simulink model "LW_ctrl_241029_1"  (R2024b)
settings: Solver=ode4  StartTime=0.0  StopTime=inf  FixedStep=0.005  RelTol=1e-3  EnableMultiTasking=on
StartFcn:
  | %timestart = cputime;
StopFcn:
  | %dt = cputime - timestart
undefined symbols (not defined in the file or in its folder): AttCtrl_cycle, ControlMode, DEG2RAD, Earth, FlightMode, LW_ACRO_P_MAX, LW_ACRO_R_MAX, LW_ACRO_Y_MAX, LW_AERO_C0, LW_AERO_C1, LW_AERO_Y0, LW_ANGLE, LW_DMZ0, LW_DMZ_MIN, LW_LAT_CIRCLE, LW_MAN_PITCH_MAX, LW_MAN_ROLL_MAX, LW_MASS, LW_OB_CIRCLE_R, LW_OB_CIRCLE_V, LW_OB_CIRCLE_W, LW_OB_TYPE, LW_REX_YAW, LW_SERVOL_MAX, LW_SERVOR_MAX, LW_TEST_DTXY, LW_TEST_DTZ, LW_THR_HOVER, LW_WZ_MAX, LW_X_ACCEL_MAX, LW_X_ACCEL_MIN, LW_X_FF, LW_X_JERK_MAX, LW_X_P, LW_X_VEL_MAX, LW_Y_ACCEL_MAX, LW_Y_ACCEL_MIN, LW_Y_FF, LW_Y_JERK_MAX, LW_Y_P, LW_Y_VEL_MAX, LW_YAW_KAD, LW_YAW_KAP, LW_Z_ACCEL_LOW, LW_Z_ACCEL_UP, LW_Z_FF, LW_Z_JERK_MAX, LW_Z_P, LW_Z_VEL_MAX_UP, Map_xoffset, Map_yoffset, Map_zoffset, MAX_wdotx, MAX_wdoty, MAX_wdotz, Mixer_cycle, ModelParam_AccelMax, ModelParam_DelayAtt, ModelParam_DelayOmega, ModelParam_DelayPos ... (+59)
libraries: pixhawk_slib_uORB_RW x15, simulink x7, slpidlib x6, dspfdesign x6, dspstat3 x5, aerolibnav x4, pixhawk_slib_sensors_actuators x3, aerolibtransform2 x3, etargetslib x2, pixhawk_slib_rfly x1, aerolibatmos2 x1, slrealtimeiplib x1
(part 4 of 6)

== system LW_ctrl_241029_1/Output/OutputSelect/Sim/Lifting Body Airframe/Estimator/Subsystem ==
  vehicle_states : Inport
  environment_states : Inport  Port=2
  Bus Selector : BusSelector  OutputSignals=Pe,Ve,wb,Vb,DCMeb,Euler,q,Ab,Abe,dwb
  Bus Selector1 : BusSelector  OutputSignals=terrainZ,landed,mag_e,mag_dec,gravity,tempcC,airPressure,altitude,airDensity,alpha,beta,airspeed,vw_e,qbar
  Transpose : Math  Operator=transpose  SignedPower=on
  Bus Element Out : Outport  PortName=Kinematics 6DOF Bus  Element=Ve
  Out Bus Element : Outport  PortName=Kinematics 6DOF Bus  Element=Xe
  Out Bus Element1 : Outport  PortName=Kinematics 6DOF Bus  Element=Euler
  Out Bus Element2 : Outport  PortName=Kinematics 6DOF Bus  Element=DCM
  Out Bus Element3 : Outport  PortName=Kinematics 6DOF Bus  Element=Vb
  Out Bus Element4 : Outport  PortName=Kinematics 6DOF Bus  Element=Wb
  Out Bus Element6 : Outport  PortName=Kinematics 6DOF Bus  Element=Abb
  Out Bus Element8 : Outport  VectorParamsAs1DForOutWhenUnconnected=off  PortName=Kinematics 6DOF Bus  Element=Quat
  Out Bus Element20 : Outport  PortName=Kinematics 6DOF Bus  Element=Abe
  Out Bus Element21 : Outport  PortName=Kinematics 6DOF Bus  Element=dWb
  Out Bus Element5 : Outport  Port=2  PortName=Environment Model Bus  Element=mag_e
  Out Bus Element7 : Outport  Port=2  PortName=Environment Model Bus  Element=mag_dec
  Out Bus Element9 : Outport  Port=2  PortName=Environment Model Bus  Element=Altitude
  Out Bus Element10 : Outport  Port=2  PortName=Environment Model Bus  Element=landed
  Out Bus Element11 : Outport  Port=2  PortName=Environment Model Bus  Element=TempC
  Out Bus Element12 : Outport  Port=2  PortName=Environment Model Bus  Element=Vwg
  Out Bus Element13 : Outport  Port=2  PortName=Environment Model Bus  Element=AirPressure
  Out Bus Element14 : Outport  Port=2  PortName=Environment Model Bus  Element=Rho
  Out Bus Element15 : Outport  Port=2  PortName=Environment Model Bus  Element=g
  Out Bus Element16 : Outport  Port=2  PortName=Environment Model Bus  Element=alpha
  Out Bus Element17 : Outport  Port=2  PortName=Environment Model Bus  Element=beta
  Out Bus Element18 : Outport  Port=2  PortName=Environment Model Bus  Element=airspeed
  Out Bus Element19 : Outport  Port=2  PortName=Environment Model Bus  Element=qbar
  Out Bus Element22 : Outport  Port=2  PortName=Environment Model Bus  Element=TerrainZ
  wires:
  Transpose/1 -> Out Bus Element2/1
  Bus Selector1/1 -> Out Bus Element22/1  "<terrainZ>"
  Bus Selector/10 -> Out Bus Element21/1  "<dwb>"
  Bus Selector/9 -> Out Bus Element20/1  "<Abe>"
  Bus Selector1/14 -> Out Bus Element19/1  "<qbar>"
  Bus Selector1/13 -> Out Bus Element12/1  "<vw_e>"
  Bus Selector1/12 -> Out Bus Element18/1  "<airspeed>"
  Bus Selector1/11 -> Out Bus Element17/1  "<beta>"
  Bus Selector1/10 -> Out Bus Element16/1  "<alpha>"
  Bus Selector1/9 -> Out Bus Element14/1  "<airDensity>"
  Bus Selector1/8 -> Out Bus Element9/1  "<altitude>"
  Bus Selector1/6 -> Out Bus Element11/1  "<tempcC>"
  Bus Selector1/7 -> Out Bus Element13/1  "<airPressure>"
  Bus Selector1/5 -> Out Bus Element15/1  "<gravity>"
  Bus Selector1/4 -> Out Bus Element7/1  "<mag_dec>"
  Bus Selector1/3 -> Out Bus Element5/1  "<mag_e>"
  Bus Selector1/2 -> Out Bus Element10/1  "<landed>"
  environment_states/1 -> Bus Selector1/1
  Bus Selector/8 -> Out Bus Element6/1  "<Ab>"
  Bus Selector/7 -> Out Bus Element8/1  "<q>"
  Bus Selector/6 -> Out Bus Element1/1  "<Euler>"
  Bus Selector/5 -> Transpose/1  "<DCMeb>"
  Bus Selector/4 -> Out Bus Element3/1  "<Vb>"
  Bus Selector/3 -> Out Bus Element4/1  "<wb>"
  Bus Selector/2 -> Bus Element Out/1  "<Ve>"
  Bus Selector/1 -> Out Bus Element/1  "<Pe>"
  vehicle_states/1 -> Bus Selector/1

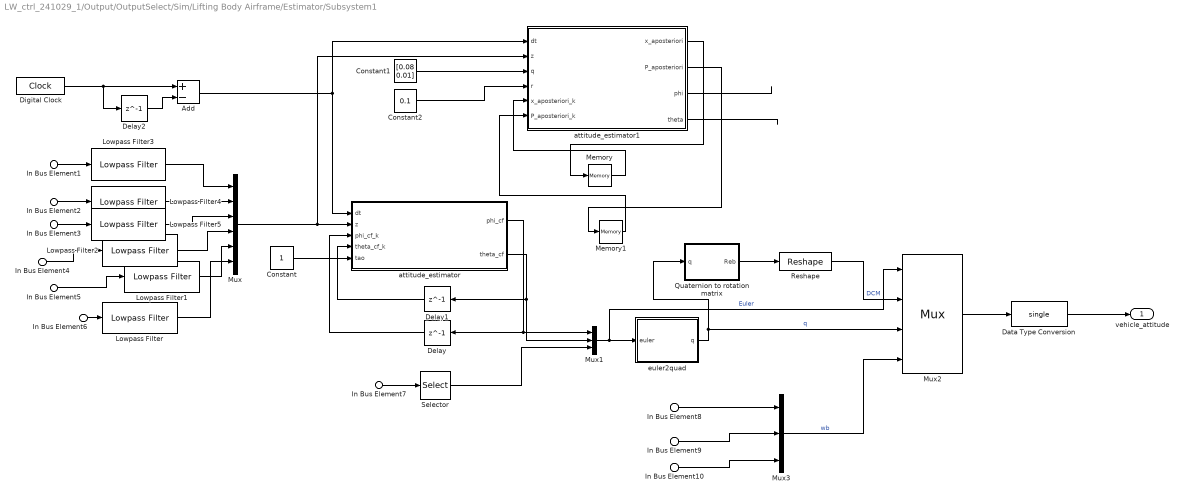
== system LW_ctrl_241029_1/Output/OutputSelect/Sim/Lifting Body Airframe/Estimator/Subsystem1 ==
  In Bus Element1 : Inport  PortName=SensorData  Element=xgyro
  In Bus Element8 : Inport  PortName=SensorData  Element=xgyro
  In Bus Element2 : Inport  PortName=SensorData  Element=ygyro
  In Bus Element9 : Inport  PortName=SensorData  Element=ygyro
  In Bus Element3 : Inport  PortName=SensorData  Element=zgyro
  In Bus Element10 : Inport  PortName=SensorData  Element=zgyro
  In Bus Element4 : Inport  PortName=SensorData  Element=xacc
  In Bus Element5 : Inport  PortName=SensorData  Element=yacc
  In Bus Element6 : Inport  PortName=SensorData  Element=zacc
  In Bus Element7 : Inport  Port=2  PortName=Kinematics 6DOF Bus  Element=Euler
  Add : Sum  Inputs=+-
  Constant : Constant
  Constant1 : Constant  Value=[0.08 0.01]
  Constant2 : Constant  Value=0.1
  Data Type Conversion : DataTypeConversion  OutDataTypeStr=single  SaturateOnIntegerOverflow=off  RndMeth=Floor
  Delay : Delay  DelayLength=1  InitialCondition=0
  Delay1 : Delay  DelayLength=1  InitialCondition=0
  Delay2 : Delay  DelayLength=1  InitialCondition=0
  Digital Clock : DigitalClock  SampleTime=0.001
  Lowpass Filter{,1..5} (6 alike) : dspfdesign/Lowpass Filter  FilterType=FIR  DesignForMinimumOrder=on  FilterOrder=50  PassbandFrequency=10  StopbandFrequency=40  PassbandRipple=0.1  StopbandAttenuation=80  SampleRateMode=Specify on dialog  SampleRate=1000  SimulateUsing=Interpreted execution  roundingMode=Floor  coeffsDataTypeStr=fixdt(1,16)
  Memory : Memory  InitialCondition=[0, 0, 0, 0, 0, -1]
  Memory1 : Memory  InitialCondition=eye(6, 6)*100
  Mux : Mux  Inputs=6
  Mux1 : Mux  Inputs=3
  Mux2 : Mux
      settings: DisplayOption=signals
  Mux3 : Mux  Inputs=3
  Quaternion to rotation matrix : MATLAB Function
  Reshape : Reshape
  Selector : Selector  InputPortWidth=3  IndexOptions=Index vector (dialog)  Indices=[ 3]  OutputSizes=1
  attitude_estimator : MATLAB Function  TreatAsAtomicUnit=on
  attitude_estimator1 : MATLAB Function  TreatAsAtomicUnit=on
  euler2quad : MATLAB Function
  vehicle_attitude : Outport
  wires:
  Constant/1 -> attitude_estimator/5(tao)
  Delay1/1 -> attitude_estimator/4(theta_cf_k)
  Delay/1 -> attitude_estimator/3(phi_cf_k)
  Mux/1 -> attitude_estimator1/2(z), attitude_estimator/2(z)
  In Bus Element1/1 -> Lowpass Filter3/1
  In Bus Element2/1 -> Lowpass Filter4/1
  In Bus Element3/1 -> Lowpass Filter5/1
  In Bus Element4/1 -> Lowpass Filter2/1
  In Bus Element5/1 -> Lowpass Filter1/1
  In Bus Element6/1 -> Lowpass Filter/1
  attitude_estimator/1(phi_cf) -> Mux1/1, Delay/1
  attitude_estimator/2(theta_cf) -> Mux1/2, Delay1/1
  Digital Clock/1 -> Add/1, Delay2/1
  Delay2/1 -> Add/2
  Add/1 -> attitude_estimator/1(dt), attitude_estimator1/1(dt)
  In Bus Element7/1 -> Selector/1
  Selector/1 -> Mux1/3
  Mux1/1 -> Mux2/1, euler2quad/1(euler)  "Euler"
  euler2quad/1(q) -> Quaternion to rotation matrix/1(q), Mux2/3  "q"
  Quaternion to rotation matrix/1(Reb) -> Reshape/1
  Reshape/1 -> Mux2/2  "DCM"
  In Bus Element8/1 -> Mux3/1
  In Bus Element9/1 -> Mux3/2
  In Bus Element10/1 -> Mux3/3
  Mux3/1 -> Mux2/4  "wb"
  Mux2/1 -> Data Type Conversion/1
  Data Type Conversion/1 -> vehicle_attitude/1
  attitude_estimator1/1(x_aposteriori) -> Memory/1
  Memory/1 -> attitude_estimator1/5(x_aposteriori_k)
  attitude_estimator1/2(P_aposteriori) -> Memory1/1
  Memory1/1 -> attitude_estimator1/6(P_aposteriori_k)
  attitude_estimator1/3(phi) -> ?
  attitude_estimator1/4(theta) -> ?
  Constant1/1 -> attitude_estimator1/3(q)
  Constant2/1 -> attitude_estimator1/4(r)
  Lowpass Filter/1 -> Mux/6
  Lowpass Filter1/1 -> Mux/5
  Lowpass Filter2/1 -> Mux/4
  Lowpass Filter3/1 -> Mux/1
  Lowpass Filter4/1 -> Mux/2
  Lowpass Filter5/1 -> Mux/3

== system LW_ctrl_241029_1/Output/OutputSelect/Sim/Lifting Body Airframe/Estimator/Subsystem2 ==
  In Bus Element1 : Inport  PortName=SensorData  Element=xgyro
  In Bus Element2 : Inport  PortName=SensorData  Element=ygyro
  In Bus Element3 : Inport  PortName=SensorData  Element=zgyro
  In Bus Element4 : Inport  PortName=SensorData  Element=xacc
  In Bus Element5 : Inport  PortName=SensorData  Element=yacc
  In Bus Element6 : Inport  PortName=SensorData  Element=zacc
  Data Type Conversion : DataTypeConversion  OutDataTypeStr=single  SaturateOnIntegerOverflow=off  RndMeth=Floor
  Mux : Mux  Inputs=6
  imu : Outport
  wires:
  In Bus Element3/1 -> Mux/3
  In Bus Element2/1 -> Mux/2
  In Bus Element1/1 -> Mux/1
  In Bus Element4/1 -> Mux/4
  In Bus Element5/1 -> Mux/5
  In Bus Element6/1 -> Mux/6
  Data Type Conversion/1 -> imu/1
  Mux/1 -> Data Type Conversion/1

== system LW_ctrl_241029_1/Output/OutputSelect/Sim/Lifting Body Airframe/To Unreal/pack ==
  note: struct SOut2Simulator
      | {
      | int copterID; //飞机ID
      | int vehicleType; //飞机构型
      | double runnedTime; //仿真时间
      | float VelE[3]; //NED地球系速度
      | float PosE[3]; //NED地球系位置
      | float AngEuler[3]; //欧拉角
      | float AngQuatern[4]; //四元数
      | float MotorRPMS[8]; //电机转速RPM
      | float AccB[3]; //机体轴加速度
      | float RateB[3]; //机体轴角速度
      | double PosGPS[3]; //地球GPS经纬高
      | }
      |
      | //SOut2Simulator的定义与Simulink里面新加的MavVehileInfo结构体完全一致
      | //可以直接对新的simulink模型的MavVehile3DInfo输出口数据进行打包
      | //两个结构体的长度都是152
      | sizeof(SOut2Simulator) = sizeof(MavVehileInfo) = 152
      |
      | 打包封装的结构体为
      | typedef struct _netDataShort
      | {
      | TargetType tg; //这里目前随便填，写1即可 uint32
      | int len; //这个长度为传输结构体长度，目前是152
      | char payload[192]; //这里面前152位存放了SOut2Simulator结构体数据，后面的40位保留
      | }netDataShort;
      |
      | //UDP包的总长度为200
      | sizeof(netDataShort) = 200
      |
      | //发送的UDP端口号为：20010
  copterID : Inport  PortDimensions=1
  vehicleType : Inport  Port=2  PortDimensions=1
  runnedTime : Inport  Port=3  PortDimensions=1
  "VelE " : Inport  Port=4  PortDimensions=3
  PosE : Inport  Port=5  PortDimensions=3
  AngEuler : Inport  Port=6  PortDimensions=3
  AngQuatern : Inport  Port=7  PortDimensions=4
  MotorRPMS : Inport  Port=8  PortDimensions=8
  AccB : Inport  Port=9  PortDimensions=3
  RateB : Inport  Port=10  PortDimensions=3
  PosGPS : Inport  Port=11  PortDimensions=3
  Data Type Conversion : DataTypeConversion  OutDataTypeStr=uint32  SaturateOnIntegerOverflow=off  RndMeth=Floor
  Data Type Conversion1 : DataTypeConversion  OutDataTypeStr=int32  SaturateOnIntegerOverflow=off  RndMeth=Floor
  Data Type Conversion2 : DataTypeConversion  OutDataTypeStr=int32  SaturateOnIntegerOverflow=off  RndMeth=Floor
  Data Type Conversion3 : DataTypeConversion  OutDataTypeStr=int32  SaturateOnIntegerOverflow=off  RndMeth=Floor
  Data Type Conversion4 : DataTypeConversion  OutDataTypeStr=double  SaturateOnIntegerOverflow=off  RndMeth=Floor
  Data Type Conversion5 : DataTypeConversion  OutDataTypeStr=single  SaturateOnIntegerOverflow=off  RndMeth=Floor
  Data Type Conversion6 : DataTypeConversion  OutDataTypeStr=double  SaturateOnIntegerOverflow=off  RndMeth=Floor
  Data Type Conversion7 : DataTypeConversion  OutDataTypeStr=double  SaturateOnIntegerOverflow=off  RndMeth=Floor
  Mux : Mux  Inputs=2
  Mux1 : Mux  Inputs=7
  Mux2 : Mux  Inputs=2
  Package Head : etargetslib/Byte Pack  datatypes={'uint32','int32'}  byteAlign=4
  PayLoad : etargetslib/Byte Pack  datatypes={'int32','double','single','double','double'}  byteAlign=8
  TargetType : Constant  OutDataTypeStr=Inherit: Inherit via back propagation
  len : Constant  Value=152  OutDataTypeStr=Inherit: Inherit via back propagation
  reserve : Constant  Value=[0 0 0 0 0]  OutDataTypeStr=double
  toUnReal : Outport  VectorParamsAs1DForOutWhenUnconnected=off
  wires:
  Data Type Conversion7/1 -> PayLoad/5
  Data Type Conversion4/1 -> PayLoad/2
  Data Type Conversion3/1 -> Mux2/2
  Data Type Conversion/1 -> Package Head/1
  Data Type Conversion6/1 -> PayLoad/4
  Data Type Conversion1/1 -> Package Head/2
  Data Type Conversion2/1 -> Mux2/1
  Data Type Conversion5/1 -> PayLoad/3
  AngEuler/1 -> Mux1/3
  Mux2/1 -> PayLoad/1
  reserve/1 -> Data Type Conversion7/1
  TargetType/1 -> Data Type Conversion/1
  PosE/1 -> Mux1/2
  vehicleType/1 -> Data Type Conversion3/1
  len/1 -> Data Type Conversion1/1
  copterID/1 -> Data Type Conversion2/1
  AngQuatern/1 -> Mux1/4
  MotorRPMS/1 -> Mux1/5
  Mux/1 -> toUnReal/1
  AccB/1 -> Mux1/6
  Package Head/1 -> Mux/1
  PosGPS/1 -> Data Type Conversion6/1
  Mux1/1 -> Data Type Conversion5/1
  "VelE "/1 -> Mux1/1
  PayLoad/1 -> Mux/2
  RateB/1 -> Mux1/7
  runnedTime/1 -> Data Type Conversion4/1

== system LW_ctrl_241029_1/rc_receive/manual_ctrl_in/Sim/Simulate ref/commandMapping/command2pwm ==
  rates_ref : Inport
  ctrl_mode : Inport  Port=2
  euler_ref : Inport  Port=3
  vel_ref : Inport  Port=4
  throttle : Inport  Port=5
  delta : Inport  Port=6
  Merge : Merge  Inputs=5
  Switch Case : SwitchCase  CaseConditions={ControlMode.MANUAL,ControlMode.ACRO, ControlMode.STABILIZED, ControlMode.ALTITUDE,ControlMode.POSITION}
  Terminator : Terminator
  acro : Subsystem  TreatAsAtomicUnit=on
  altitude : Subsystem  TreatAsAtomicUnit=on
  euler_ref1 : InportShadow  Port=3
  man : Subsystem  TreatAsAtomicUnit=on
  position : Subsystem  TreatAsAtomicUnit=on
  rates_r_ref : InportShadow
  rates_r_ref1 : InportShadow
  rates_r_ref2 : InportShadow
  stabilized : Subsystem  TreatAsAtomicUnit=on
  throttle1 : InportShadow  Port=5
  vel_ref1 : InportShadow  Port=4
  manual_ref : Outport
  wires:
  Switch Case/4 -> altitude/Action
  Switch Case/3 -> stabilized/Action
  ctrl_mode/1 -> Switch Case/1
  rates_ref/1 -> acro/1(rc_input)
  altitude/1(altitude_ref) -> Merge/4
  Switch Case/2 -> acro/Action
  stabilized/1(stabilizd_ref) -> Merge/3
  Switch Case/5 -> position/Action
  throttle/1 -> acro/2(throttle)
  euler_ref/1 -> stabilized/1(euler_ref)
  throttle1/1 -> stabilized/2(throttle)
  vel_ref/1 -> altitude/3(vel_ref)
  rates_r_ref/1 -> stabilized/3(rates_r_ref)
  rates_r_ref1/1 -> altitude/2(rates_r_ref)
  vel_ref1/1 -> position/1(vel_ref)
  rates_r_ref2/1 -> position/2(rates_r_ref)
  euler_ref1/1 -> altitude/1(euler_ref)
  position/1(position_ref) -> Merge/5
  acro/1(acro_ref) -> Merge/2
  Switch Case/6 -> Terminator/1
  Merge/1 -> manual_ref/1
  delta/1 -> man/1(delta)
  Switch Case/1 -> man/Action
  man/1(delta_ref) -> Merge/1

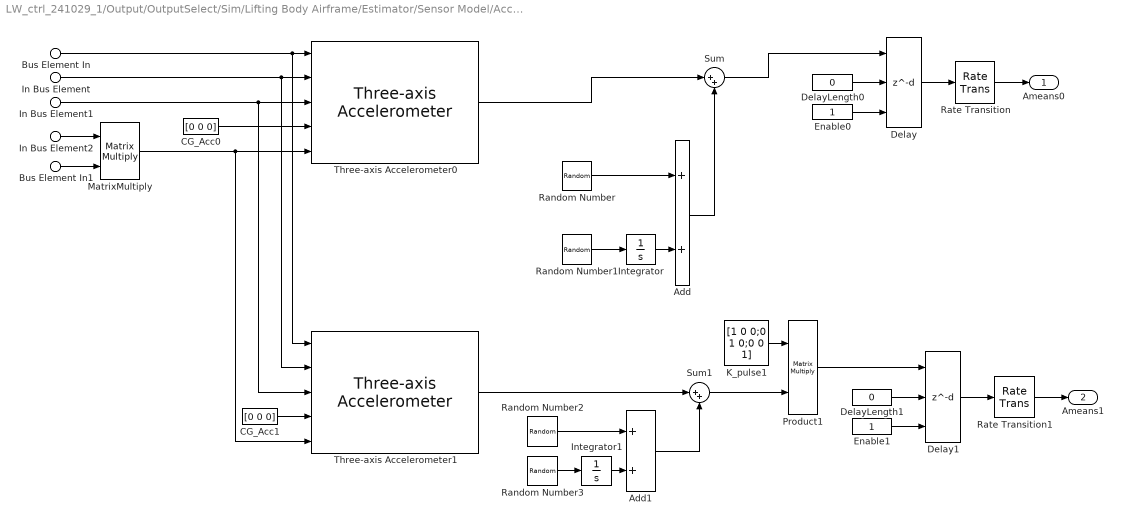
== system LW_ctrl_241029_1/Output/OutputSelect/Sim/Lifting Body Airframe/Estimator/Sensor Model/Accelerometer Hub ==
  Bus Element In1 : Inport  PortName=Environment Model Bus  Element=g
  Bus Element In : Inport  Port=2  PortName=Kinematics 6DOF Bus  Element=Abe
  In Bus Element : Inport  Port=2  PortName=Kinematics 6DOF Bus  Element=Wb
  In Bus Element1 : Inport  Port=2  PortName=Kinematics 6DOF Bus  Element=dWb
  In Bus Element2 : Inport  Port=2  PortName=Kinematics 6DOF Bus  Element=DCM
  Add : Sum
  Add1 : Sum
  CG_Acc0 : Constant  Value=[0 0 0]
  CG_Acc1 : Constant  Value=[0 0 0]
  Delay : Delay  DelayLengthSource=Input port  ShowEnablePort=on
      settings: InputPortMap=u0,p1,e6
  Delay1 : Delay  DelayLengthSource=Input port  ShowEnablePort=on
      settings: InputPortMap=u0,p1,e6
  DelayLength0 : Constant  Value=0
  DelayLength1 : Constant  Value=0
  Enable0 : Constant
  Enable1 : Constant
  Integrator : Integrator
  Integrator1 : Integrator
  K_pulse1 : Constant  Value=[1 0 0;0 1 0;0 0 1]
  MatrixMultiply : Product  Multiplication=Matrix(*)
  Product1 : Product  Multiplication=Matrix(*)
  Random Number : RandomNumber  Variance=ModelParam_noiseAccelNa  Seed=ModelParam_noiseAccelNaSeed  SampleTime=0.004
  Random Number1 : RandomNumber  Variance=ModelParam_noiseAccelBa  Seed=ModelParam_noiseAccelBaSeed  SampleTime=0.004
  Random Number2 : RandomNumber  Mean=[0 0 0]  Variance=[0.1 0.1 0.1]  Seed=[235 341 569]  SampleTime=SampleTime
  Random Number3 : RandomNumber  Mean=[0 0 0]  Variance=[0.1 0.1 0.1]  Seed=[3341 365 597]  SampleTime=SampleTime
  Rate Transition : RateTransition
  Rate Transition1 : RateTransition
  Sum : Sum  Inputs=|++
  Sum1 : Sum  Inputs=|++
  Three-axis Accelerometer0 : aerolibnav/Three-axis Accelerometer  units=Metric (MKS)  acc=[0 0 0]  gtype=on  dtype_a=on  w_a=190  z_a=0.707  a_sf_cc=[1 0 0; 0 1 0; 0 0 1]  a_bias=[0 0 0]  a_Ts=0  a_rand=off  a_seeds=[23093 23094 23095]  a_pow=[0.001 0.001 0.001]  a_sat="[-inf  -inf  -inf  inf inf inf]"
  Three-axis Accelerometer1 : aerolibnav/Three-axis Accelerometer  units=Metric (MKS)  acc=[0 0 0]  gtype=on  dtype_a=on  w_a=190  z_a=0.707  a_sf_cc=[1 0 0; 0 1 0; 0 0 1]  a_bias=[0 0 0]  a_Ts=0  a_rand=off  a_seeds=[23093 23094 23095]  a_pow=[0.001 0.001 0.001]  a_sat="[-inf  -inf  -inf  inf inf inf]"
  Ameans0 : Outport
  Ameans1 : Outport  Port=2
  wires:
  Add/1 -> Sum/2
  Random Number1/1 -> Integrator/1
  Random Number/1 -> Add/1
  Three-axis Accelerometer0/1 -> Sum/1
  K_pulse1/1 -> Product1/1
  Product1/1 -> Delay1/1
  Sum/1 -> Delay/1
  Random Number2/1 -> Add1/1
  Integrator1/1 -> Add1/2
  Random Number3/1 -> Integrator1/1
  Add1/1 -> Sum1/2
  Sum1/1 -> Product1/2
  Integrator/1 -> Add/2
  In Bus Element2/1 -> MatrixMultiply/1
  Bus Element In/1 -> Three-axis Accelerometer0/1, Three-axis Accelerometer1/1
  In Bus Element/1 -> Three-axis Accelerometer0/2, Three-axis Accelerometer1/2
  Bus Element In1/1 -> MatrixMultiply/2
  In Bus Element1/1 -> Three-axis Accelerometer1/3, Three-axis Accelerometer0/3
  Delay1/1 -> Rate Transition1/1
  Three-axis Accelerometer1/1 -> Sum1/1
  Rate Transition1/1 -> Ameans1/1
  Enable1/1 -> Delay1/3
  DelayLength1/1 -> Delay1/2
  DelayLength0/1 -> Delay/2
  Enable0/1 -> Delay/3
  Rate Transition/1 -> Ameans0/1
  CG_Acc0/1 -> Three-axis Accelerometer0/4
  Delay/1 -> Rate Transition/1
  CG_Acc1/1 -> Three-axis Accelerometer1/4
  MatrixMultiply/1 -> Three-axis Accelerometer0/5, Three-axis Accelerometer1/5

== system LW_ctrl_241029_1/Output/OutputSelect/Sim/Lifting Body Airframe/Estimator/Sensor Model/Barometer ==
  In Bus Element : Inport  PortName=Environment Model Bus  Element=Altitude
  In Bus Element2 : Inport  PortName=Environment Model Bus  Element=TempC
  In Bus Element1 : Inport  PortName=Environment Model Bus  Element=qbar
  Add2 : Sum
  Gain : Gain  Gain=0.01
  Gain3 : Gain  Gain=0.01
  ISA Atmosphere Model : aerolibatmos2/ISA Atmosphere Model  useExtended=off  action=Warning  custom=off  viscosityOut=off  g=9.80665  gamma=1.4  R=287.0531  L=0.0065  h_trop=11000  h_strat=20000  rho0=1.225  P0=101325  T0=288.15  h0=0  S=110.4  Tref=273.15  muref=1.716e-5
  Integrator1 : Integrator
  K_pulse0 : Constant
  Product : Product
  Random Number1 : RandomNumber  Variance=ModelParam_noiseBaroNm  Seed=ModelParam_noiseBaroNmSeed  SampleTime=0.004
  Random Number2 : RandomNumber  Variance=ModelParam_noiseBaroNbm  Seed=ModelParam_noiseBaroNbmSeed  SampleTime=0.004
  Sum : Sum  Inputs=|++
  Terminator : Terminator
  Terminator1 : Terminator
  Terminator2 : Terminator
  Pressure : Outport
  diff_pressure : Outport  Port=2
  pressure_alt : Outport  Port=3  PortDimensions=1
  temperature : Outport  Port=4
  wires:
  In Bus Element1/1 -> Gain/1
  ISA Atmosphere Model/4 -> Terminator2/1
  ISA Atmosphere Model/2 -> Terminator1/1
  ISA Atmosphere Model/1 -> Terminator/1
  Random Number2/1 -> Integrator1/1
  Add2/1 -> Sum/2
  Random Number1/1 -> Add2/1
  Integrator1/1 -> Add2/2
  Gain3/1 -> Pressure/1
  Gain/1 -> diff_pressure/1
  In Bus Element2/1 -> temperature/1
  ISA Atmosphere Model/3 -> Gain3/1
  K_pulse0/1 -> Product/1
  Sum/1 -> Product/2
  In Bus Element/1 -> Sum/1
  Product/1 -> pressure_alt/1, ISA Atmosphere Model/1

== system LW_ctrl_241029_1/Output/OutputSelect/Sim/Lifting Body Airframe/Estimator/Sensor Model/GPS ==
  In Bus Element : Inport  PortName=Kinematics 6DOF Bus  Element=Xe
  In Bus Element1 : Inport  PortName=Kinematics 6DOF Bus  Element=Ve
  In Bus Element2 : Inport  PortName=Kinematics 6DOF Bus  Element=Euler
  -pi-pi---->0-2pi : MATLAB Function  TreatAsAtomicUnit=on
  BiasGain1 : Gain  Gain=0.1
  Demux : Demux  Outputs=3
  Demux1 : Demux  Outputs=3
  Flat Earth to LLA : aerolibtransform2/Flat Earth to LLA  units=Metric (MKS)  ptype=Earth (WGS84)  F=1/298.257223563  R=6378137  refPosPort=off  LL0=ModelParam_GPSLatLong  psi=0
  Gain1 : Gain  Gain=0.2*0.58
  GenCogVel : MATLAB Function  TreatAsAtomicUnit=on
  ModelParam.GPSEphFinal : Constant  Value=ModelParam_GPSEphFinal
  ModelParam.GPSEpvFinal : Constant  Value=ModelParam_GPSEpvFinal
  ModelParam.GPSSatsVisible : Constant  Value=ModelParam_GPSSatsVisible
  ModelParam_GPSFix3DFix : Constant  Value=ModelParam_GPSFix3DFix
  ModelParam_envAltitude : Constant  Value=ModelParam_envAltitude
  Mux : Mux  Inputs=2
  Mux1 : Mux  Inputs=13
  NoiseFilter1 : Subsystem
  Saturation : Saturate  UpperLimit=100000  LowerLimit=0
  Selector : Selector  InputPortWidth=3  IndexOptions=Index vector (dialog)  Indices=[3]  OutputSizes=1
  Sum : Sum  Inputs=|++
  Sum3 : Sum  Inputs=|++
  Uniform Random Number1 : UniformRandomNumber  Minimum=[-1,-1,-2]  Maximum=[1,1,2]  Seed=[1452,787,69]  SampleTime=ModelParam_noiseGPSSampTime
  Uniform Random Number4 : UniformRandomNumber  Minimum=[-1,-1,-2]  Maximum=[1,1,2]  Seed=[5445,45433,33433]  SampleTime=ModelParam_noiseGPSSampTime
  GPS : Outport
  wires:
  NoiseFilter1/1(Out1) -> Sum3/2
  BiasGain1/1 -> NoiseFilter1/1(In1)
  Uniform Random Number4/1 -> BiasGain1/1
  Sum3/1 -> GenCogVel/1(u), Demux1/1
  Saturation/1 -> Mux/2
  Gain1/1 -> Sum/2
  Uniform Random Number1/1 -> Gain1/1
  ModelParam.GPSSatsVisible/1 -> Mux1/12  "satellites_visible"
  ModelParam_GPSFix3DFix/1 -> Mux1/11  "fixtype"
  -pi-pi---->0-2pi/1(yaw360) -> Mux1/13  "headVeh"
  Selector/1 -> -pi-pi---->0-2pi/1(yaw180)
  In Bus Element2/1 -> Selector/1
  GenCogVel/2(cot) -> Mux1/7  "cog"
  GenCogVel/1(v) -> Mux1/6  "vel"
  Demux1/3 -> Mux1/10  "vd"
  Demux1/2 -> Mux1/9  "ve"
  Demux1/1 -> Mux1/8  "vn"
  In Bus Element1/1 -> Sum3/1
  Mux1/1 -> GPS/1
  ModelParam.GPSEpvFinal/1 -> Mux1/5  "epv"
  ModelParam.GPSEphFinal/1 -> Mux1/4  "eph"
  Demux/3 -> Mux1/3  "alt"
  Demux/1 -> Mux1/1  "lat"
  Demux/2 -> Mux1/2  "lon"
  Mux/1 -> Demux/1
  Flat Earth to LLA/2 -> Saturation/1
  Flat Earth to LLA/1 -> Mux/1
  Sum/1 -> Flat Earth to LLA/1
  In Bus Element/1 -> Sum/1
  ModelParam_envAltitude/1 -> Flat Earth to LLA/2

== system LW_ctrl_241029_1/Output/OutputSelect/Sim/Lifting Body Airframe/Estimator/Sensor Model/Gyroscope Hub ==
  In Bus Element : Inport  PortName=Kinematics 6DOF Bus  Element=Wb
  In Bus Element1 : Inport  PortName=Kinematics 6DOF Bus  Element=Abe
  Acceleration Conversion : aerolibnav/Three-axis Inertial Measurement Unit/Acceleration Conversion  SystemSampleTime=-1  VariantActivationTime=update diagram  AllowFlexibleInterface=on  Latency=0  AutoFrameSizeCalculation=off
  Add2 : Sum
  Delay : Delay  DelayLengthSource=Input port  ShowEnablePort=on
      settings: InputPortMap=u0,p1,e6
  DelayLength0 : Constant  Value=0
  Enable0 : Constant
  Integrator : Integrator
  Random Number : RandomNumber  Variance=ModelParam_noiseGyroNg  Seed=ModelParam_noiseGyroNgSeed  SampleTime=0.004
  Random Number1 : RandomNumber  Variance=ModelParam_noiseGyroNbg  Seed=ModelParam_noiseGyroNbgSeed  SampleTime=0.004
  Rate Transition : RateTransition
  Sum : Sum  Inputs=|++
  Three-axis Gyroscope0 : aerolibnav/Three-axis Gyroscope  dtype_g=on  w_g=190  z_g=0.707  g_sf_cc=[1 0 0; 0 1 0; 0 0 1]  g_bias=[0 0 0]  g_sen=[0 0 0]  g_Ts=0  g_rand=off  g_seeds=[23093 23094 23095]  g_pow=[0.0001 0.0001 0.0001]  g_sat="[-inf  -inf  -inf  inf inf inf]"
  Wmeans0 : Outport
  wires:
  Sum/1 -> Delay/1
  Random Number/1 -> Add2/1
  Add2/1 -> Sum/2
  Three-axis Gyroscope0/1 -> Sum/1
  Random Number1/1 -> Integrator/1
  Integrator/1 -> Add2/2
  DelayLength0/1 -> Delay/2
  Rate Transition/1 -> Wmeans0/1
  Delay/1 -> Rate Transition/1
  Enable0/1 -> Delay/3
  Acceleration Conversion/1 -> Three-axis Gyroscope0/2
  In Bus Element/1 -> Three-axis Gyroscope0/1
  In Bus Element1/1 -> Acceleration Conversion/1

== system LW_ctrl_241029_1/Output/OutputSelect/Sim/Lifting Body Airframe/Estimator/Sensor Model/Magnetometer Hub ==
  In Bus Element : Inport  PortName=Kinematics 6DOF Bus  Element=DCM
  In Bus Element1 : Inport  Port=2  PortName=Environment Model Bus  Element=mag_e
  In Bus Element3 : Inport  Port=2  PortName=Environment Model Bus  Element=mag_e
  Delay : Delay  DelayLengthSource=Input port  ShowEnablePort=on
      settings: InputPortMap=u0,p1,e6
  Delay1 : Delay  DelayLengthSource=Input port  ShowEnablePort=on
      settings: InputPortMap=u0,p1,e6
  DelayLength0 : Constant  Value=0
  DelayLength1 : Constant  Value=0
  Enable0 : Constant
  Enable1 : Constant
  Integrator : Integrator
  Integrator1 : Integrator
  K_m1 : Constant  Value=[1 0 0; 0 1 0; 0 0 1]
  K_m2 : Constant  Value=[1 0 0; 0 1 0; 0 0 1]
  K_pulse0 : Constant  Value=[1 0 0;0 1 0;0 0 1]
  K_pulse1 : Constant  Value=[1 0 0;0 1 0;0 0 1]
  MATLAB Function : MATLAB Function  TreatAsAtomicUnit=on
  MATLAB Function1 : MATLAB Function  TreatAsAtomicUnit=on
  Measurement bias1 : Constant  Value=[0 0 0]
  Product : Product  Multiplication=Matrix(*)
  Product1 : Product  Multiplication=Matrix(*)
  Random Number : RandomNumber  Variance=ModelParam_noiseMagNm  Seed=ModelParam_noiseMagNmSeed  SampleTime=0.004
  Random Number1 : RandomNumber  Variance=ModelParam_noiseMagNm  Seed=[45465,454534,1234232]  SampleTime=0.004
  Random Number2 : RandomNumber  Mean=[0 0 0]  Variance=[0.1 0.1 0.1]  Seed=[666 588 477]  SampleTime=0.001
  Random Number3 : RandomNumber  Mean=[0 0 0]  Variance=[0.1 0.1 0.1]  Seed=[111 222 333]  SampleTime=0.001
  Rate Transition : RateTransition
  Rate Transition1 : RateTransition
  Sum1 : Sum  Inputs=|++
  Mag_means0 : Outport
  Mag_means1 : Outport  Port=2
  wires:
  In Bus Element3/1 -> MATLAB Function1/2(mag_e)
  In Bus Element1/1 -> MATLAB Function/2(mag_e)
  Integrator/1 -> MATLAB Function/3(b_m)
  Random Number/1 -> MATLAB Function/4(n_m)
  K_m2/1 -> MATLAB Function/5(K_m)
  Measurement bias1/1 -> Sum1/2
  Sum1/1 -> MATLAB Function1/3(b_m)
  Product1/1 -> Delay1/1
  K_pulse1/1 -> Product1/1
  K_pulse0/1 -> Product/1
  Product/1 -> Delay/1
  Random Number3/1 -> Integrator1/1
  Random Number1/1 -> Integrator/1
  Rate Transition1/1 -> Mag_means1/1
  Delay1/1 -> Rate Transition1/1
  DelayLength1/1 -> Delay1/2
  Enable1/1 -> Delay1/3
  MATLAB Function1/1(Mag_means) -> Product1/2
  MATLAB Function/1(Mag_means) -> Product/2
  Enable0/1 -> Delay/3
  DelayLength0/1 -> Delay/2
  Delay/1 -> Rate Transition/1
  Rate Transition/1 -> Mag_means0/1
  Random Number2/1 -> MATLAB Function1/4(n_m)
  Integrator1/1 -> Sum1/1
  K_m1/1 -> MATLAB Function1/5(K_m)
  In Bus Element/1 -> MATLAB Function1/1(DCM), MATLAB Function/1(DCM)

== system LW_ctrl_241029_1/rc_receive/manual_ctrl_in/Sim/Simulate ref/commandMapping/command2pwm/acro ==
  rc_input : Inport
  throttle : Inport  Port=2
  Action Port : ActionPort  ActionPortLabel=case [ ACRO ]:
  Constant7 : Constant  Value=1000
  Constant8 : Constant  Value=1500
  Data Type Conversion4 : DataTypeConversion  OutDataTypeStr=single  SaturateOnIntegerOverflow=off  RndMeth=Floor
  Data Type Conversion5 : DataTypeConversion  OutDataTypeStr=single  SaturateOnIntegerOverflow=off  RndMeth=Floor
  Demux : Demux  Outputs=3
  Gain1 : Gain  Gain=1/LW_ACRO_R_MAX
  Gain10 : Gain  Gain=1/LW_ACRO_P_MAX
  Gain12 : Gain  Gain=1/LW_ACRO_Y_MAX
  Gain4 : Gain  Gain=RC1_REV
  Mux1 : Mux  Inputs=6
      settings: DisplayOption=signals
  Saturation1 : Saturate  UpperLimit=1  LowerLimit=0
  Saturation2 : Saturate  UpperLimit=1  LowerLimit=-1
  Saturation3 : Saturate  UpperLimit=1  LowerLimit=-1
  Saturation4 : Saturate  UpperLimit=1  LowerLimit=-1
  wx_deadzone_inv : MATLAB Function  TreatAsAtomicUnit=on
  wy_deadzone_inv : MATLAB Function  TreatAsAtomicUnit=on
  wz_deadzone_inv : MATLAB Function  TreatAsAtomicUnit=on
  acro_ref : Outport
  wires:
  rc_input/1 -> Demux/1
  Demux/1 -> Gain1/1
  Gain1/1 -> wy_deadzone_inv/1(u)
  Gain10/1 -> wx_deadzone_inv/1(u)
  Demux/2 -> Gain10/1
  throttle/1 -> Saturation1/1  "CH2"
  Constant7/1 -> Data Type Conversion4/1  "CH5"
  Constant8/1 -> Data Type Conversion5/1  "CH7"
  Mux1/1 -> acro_ref/1  "rc"
  Saturation2/1 -> Mux1/2  "y"
  Saturation3/1 -> Mux1/1  "x"
  Saturation1/1 -> Mux1/3  "z"
  Data Type Conversion4/1 -> Mux1/5  "CH5"
  Data Type Conversion5/1 -> Mux1/6  "CH7"
  Demux/3 -> Gain12/1
  Gain12/1 -> wz_deadzone_inv/1(u)
  wz_deadzone_inv/1(y) -> Saturation4/1
  Saturation4/1 -> Mux1/4  "r"
  wx_deadzone_inv/1(y) -> Saturation3/1
  wy_deadzone_inv/1(y) -> Gain4/1
  Gain4/1 -> Saturation2/1

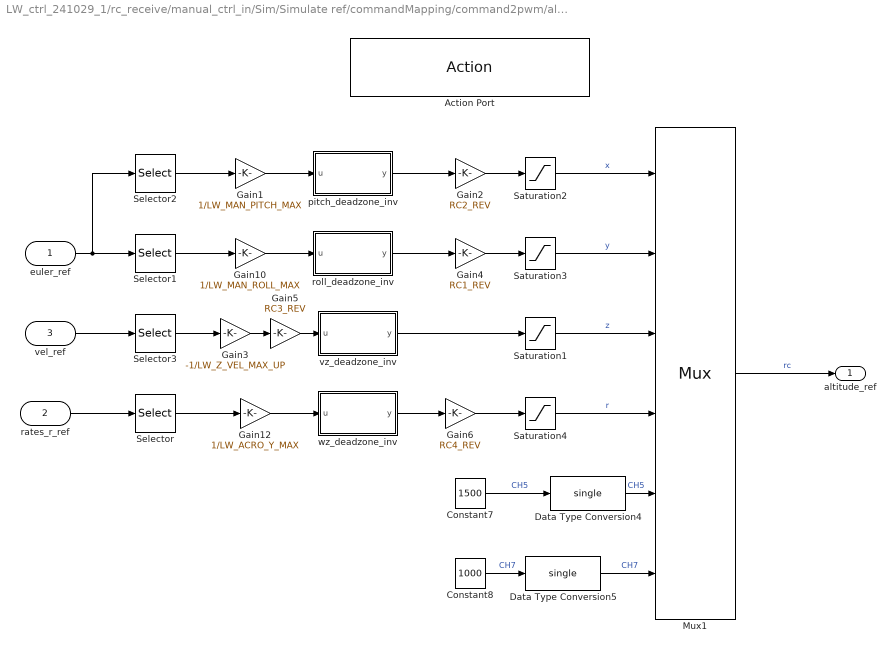
== system LW_ctrl_241029_1/rc_receive/manual_ctrl_in/Sim/Simulate ref/commandMapping/command2pwm/altitude ==
  euler_ref : Inport
  rates_r_ref : Inport  Port=2
  vel_ref : Inport  Port=3
  Action Port : ActionPort  ActionPortLabel=case [ ALTITUDE ]:
  Constant7 : Constant  Value=1500
  Constant8 : Constant  Value=1000
  Data Type Conversion4 : DataTypeConversion  OutDataTypeStr=single  SaturateOnIntegerOverflow=off  RndMeth=Floor
  Data Type Conversion5 : DataTypeConversion  OutDataTypeStr=single  SaturateOnIntegerOverflow=off  RndMeth=Floor
  Gain1 : Gain  Gain=1/LW_MAN_PITCH_MAX
  Gain10 : Gain  Gain=1/LW_MAN_ROLL_MAX
  Gain12 : Gain  Gain=1/LW_ACRO_Y_MAX
  Gain2 : Gain  Gain=RC2_REV
  Gain3 : Gain  Gain=-1/LW_Z_VEL_MAX_UP
  Gain4 : Gain  Gain=RC1_REV
  Gain5 : Gain  Gain=RC3_REV
  Gain6 : Gain  Gain=RC4_REV
  Mux1 : Mux  Inputs=6
      settings: DisplayOption=signals
  Saturation1 : Saturate  UpperLimit=1  LowerLimit=0
  Saturation2 : Saturate  UpperLimit=1  LowerLimit=-1
  Saturation3 : Saturate  UpperLimit=1  LowerLimit=-1
  Saturation4 : Saturate  UpperLimit=1  LowerLimit=-1
  Selector : Selector  InputPortWidth=3  IndexOptions=Index vector (dialog)  Indices=[ 3]  OutputSizes=1
  Selector1 : Selector  InputPortWidth=3  IndexOptions=Index vector (dialog)  Indices=1  OutputSizes=1
  Selector2 : Selector  InputPortWidth=3  IndexOptions=Index vector (dialog)  Indices=2  OutputSizes=1
  Selector3 : Selector  InputPortWidth=3  IndexOptions=Index vector (dialog)  Indices=3  OutputSizes=1
  pitch_deadzone_inv : MATLAB Function  TreatAsAtomicUnit=on
  roll_deadzone_inv : MATLAB Function  TreatAsAtomicUnit=on
  vz_deadzone_inv : MATLAB Function  TreatAsAtomicUnit=on
  wz_deadzone_inv : MATLAB Function  TreatAsAtomicUnit=on
  altitude_ref : Outport
  wires:
  Data Type Conversion4/1 -> Mux1/5  "CH5"
  Data Type Conversion5/1 -> Mux1/6  "CH7"
  Constant8/1 -> Data Type Conversion5/1  "CH7"
  Selector/1 -> Gain12/1
  Constant7/1 -> Data Type Conversion4/1  "CH5"
  rates_r_ref/1 -> Selector/1
  Mux1/1 -> altitude_ref/1  "rc"
  vel_ref/1 -> Selector3/1
  Saturation2/1 -> Mux1/1  "x"
  Saturation3/1 -> Mux1/2  "y"
  Selector2/1 -> Gain1/1
  Selector1/1 -> Gain10/1
  Gain1/1 -> pitch_deadzone_inv/1(u)
  Gain10/1 -> roll_deadzone_inv/1(u)
  euler_ref/1 -> Selector1/1, Selector2/1
  Saturation1/1 -> Mux1/3  "z"
  Gain3/1 -> Gain5/1
  Selector3/1 -> Gain3/1
  Saturation4/1 -> Mux1/4  "r"
  Gain12/1 -> wz_deadzone_inv/1(u)
  pitch_deadzone_inv/1(y) -> Gain2/1
  roll_deadzone_inv/1(y) -> Gain4/1
  wz_deadzone_inv/1(y) -> Gain6/1
  Gain2/1 -> Saturation2/1
  Gain4/1 -> Saturation3/1
  vz_deadzone_inv/1(y) -> Saturation1/1
  Gain6/1 -> Saturation4/1
  Gain5/1 -> vz_deadzone_inv/1(u)

== system LW_ctrl_241029_1/rc_receive/manual_ctrl_in/Sim/Simulate ref/commandMapping/command2pwm/man ==
  delta : Inport
  Action Port : ActionPort  ActionPortLabel=case [ MANUAL ]:
  Constant1 : Constant  Value=1000
  Constant7 : Constant  Value=1000
  Constant8 : Constant  Value=1800
  Data Type Conversion1 : DataTypeConversion  OutDataTypeStr=single  SaturateOnIntegerOverflow=off  RndMeth=Floor
  Data Type Conversion4 : DataTypeConversion  OutDataTypeStr=single  SaturateOnIntegerOverflow=off  RndMeth=Floor
  Data Type Conversion5 : DataTypeConversion  OutDataTypeStr=single  SaturateOnIntegerOverflow=off  RndMeth=Floor
  Demux : Demux  Outputs=3
  Gain1 : Gain  Gain=1/(LW_SERVOR_MAX+LW_SERVOL_MAX)
  Gain10 : Gain  Gain=1/(LW_SERVOR_MAX+LW_SERVOL_MAX)
  Gain12 : Gain  Gain=0
  Mux1 : Mux  Inputs=6
      settings: DisplayOption=signals
  Saturation2 : Saturate  UpperLimit=1  LowerLimit=-1
  Saturation3 : Saturate  UpperLimit=1  LowerLimit=-1
  Saturation4 : Saturate  UpperLimit=1  LowerLimit=-1
  delta_a_inv : MATLAB Function  TreatAsAtomicUnit=on
  delta_e_inv : MATLAB Function  TreatAsAtomicUnit=on
  delta_r_inv : MATLAB Function  TreatAsAtomicUnit=on
  delta_ref : Outport
  wires:
  delta_a_inv/1(y) -> Saturation2/1
  Saturation4/1 -> Mux1/4  "r"
  delta_r_inv/1(y) -> Saturation4/1
  Gain12/1 -> delta_r_inv/1(u)
  Demux/3 -> Gain12/1
  Data Type Conversion5/1 -> Mux1/6  "CH7"
  Data Type Conversion4/1 -> Mux1/5  "CH5"
  Saturation3/1 -> Mux1/1  "x"
  Saturation2/1 -> Mux1/2  "y"
  Mux1/1 -> delta_ref/1  "rc"
  Constant8/1 -> Data Type Conversion5/1  "CH7"
  Constant7/1 -> Data Type Conversion4/1  "CH5"
  Demux/2 -> Gain10/1
  Gain10/1 -> delta_e_inv/1(u)
  Gain1/1 -> delta_a_inv/1(u)
  Demux/1 -> Gain1/1
  delta/1 -> Demux/1
  Constant1/1 -> Data Type Conversion1/1  "z"
  Data Type Conversion1/1 -> Mux1/3  "z"
  delta_e_inv/1(y) -> Saturation3/1

== system LW_ctrl_241029_1/rc_receive/manual_ctrl_in/Sim/Simulate ref/commandMapping/command2pwm/position ==
  vel_ref : Inport
  rates_r_ref : Inport  Port=2
  Action Port : ActionPort  ActionPortLabel=case [ POSITION ]:
  Constant7 : Constant  Value=2000
  Constant8 : Constant  Value=1000
  Data Type Conversion4 : DataTypeConversion  OutDataTypeStr=single  SaturateOnIntegerOverflow=off  RndMeth=Floor
  Data Type Conversion5 : DataTypeConversion  OutDataTypeStr=single  SaturateOnIntegerOverflow=off  RndMeth=Floor
  Gain1 : Gain  Gain=-1/LW_X_VEL_MAX
  Gain10 : Gain  Gain=1/LW_Y_VEL_MAX
  Gain12 : Gain  Gain=1/LW_ACRO_Y_MAX
  Gain2 : Gain  Gain=RC2_REV
  Gain3 : Gain  Gain=-1/LW_Z_VEL_MAX_UP
  Gain4 : Gain  Gain=RC1_REV
  Gain5 : Gain  Gain=RC3_REV
  Gain6 : Gain  Gain=RC4_REV
  Mux1 : Mux  Inputs=6
      settings: DisplayOption=signals
  Saturation1 : Saturate  UpperLimit=1  LowerLimit=0
  Saturation2 : Saturate  UpperLimit=1  LowerLimit=-1
  Saturation3 : Saturate  UpperLimit=1  LowerLimit=-1
  Saturation4 : Saturate  UpperLimit=1  LowerLimit=-1
  Selector : Selector  InputPortWidth=3  IndexOptions=Index vector (dialog)  Indices=[ 3]  OutputSizes=1
  Selector1 : Selector  InputPortWidth=3  IndexOptions=Index vector (dialog)  Indices=2  OutputSizes=1
  Selector2 : Selector  InputPortWidth=3  IndexOptions=Index vector (dialog)  Indices=1  OutputSizes=1
  Selector3 : Selector  InputPortWidth=3  IndexOptions=Index vector (dialog)  Indices=3  OutputSizes=1
  vx_deadzone_inv : MATLAB Function  TreatAsAtomicUnit=on
  vy_deadzone_inv : MATLAB Function  TreatAsAtomicUnit=on
  vz_deadzone_inv : MATLAB Function  TreatAsAtomicUnit=on
  wz_deadzone_inv : MATLAB Function  TreatAsAtomicUnit=on
  position_ref : Outport
  wires:
  Mux1/1 -> position_ref/1  "rc"
  rates_r_ref/1 -> Selector/1
  Saturation3/1 -> Mux1/2  "y"
  vel_ref/1 -> Selector3/1, Selector2/1, Selector1/1
  Selector1/1 -> Gain10/1
  Gain1/1 -> vx_deadzone_inv/1(u)
  Data Type Conversion5/1 -> Mux1/6  "CH7"
  Gain10/1 -> vy_deadzone_inv/1(u)
  Data Type Conversion4/1 -> Mux1/5  "CH5"
  Selector2/1 -> Gain1/1
  Saturation2/1 -> Mux1/1  "x"
  Saturation4/1 -> Mux1/4  "r"
  Constant8/1 -> Data Type Conversion5/1
  Constant7/1 -> Data Type Conversion4/1
  Gain12/1 -> wz_deadzone_inv/1(u)
  Selector/1 -> Gain12/1
  wz_deadzone_inv/1(y) -> Gain6/1
  vy_deadzone_inv/1(y) -> Gain4/1
  vx_deadzone_inv/1(y) -> Gain2/1
  Gain2/1 -> Saturation2/1
  Gain4/1 -> Saturation3/1
  Gain6/1 -> Saturation4/1
  Gain3/1 -> Gain5/1
  vz_deadzone_inv/1(y) -> Saturation1/1
  Selector3/1 -> Gain3/1
  Saturation1/1 -> Mux1/3  "z"
  Gain5/1 -> vz_deadzone_inv/1(u)

== system LW_ctrl_241029_1/rc_receive/manual_ctrl_in/Sim/Simulate ref/commandMapping/command2pwm/stabilized ==
  euler_ref : Inport
  throttle : Inport  Port=2
  rates_r_ref : Inport  Port=3
  Action Port : ActionPort  ActionPortLabel=case [ STABILIZED ]:
  Constant7 : Constant  Value=1000
  Constant8 : Constant  Value=1000
  Data Type Conversion4 : DataTypeConversion  OutDataTypeStr=single  SaturateOnIntegerOverflow=off  RndMeth=Floor
  Data Type Conversion5 : DataTypeConversion  OutDataTypeStr=single  SaturateOnIntegerOverflow=off  RndMeth=Floor
  Gain1 : Gain  Gain=1/LW_MAN_PITCH_MAX
  Gain10 : Gain  Gain=1/LW_MAN_ROLL_MAX
  Gain12 : Gain  Gain=1/LW_WZ_MAX
  Gain4 : Gain  Gain=RC2_REV
  Mux1 : Mux  Inputs=6
      settings: DisplayOption=signals
  Saturation1 : Saturate  UpperLimit=1  LowerLimit=0
  Saturation2 : Saturate  UpperLimit=1  LowerLimit=-1
  Saturation3 : Saturate  UpperLimit=1  LowerLimit=-1
  Saturation4 : Saturate  UpperLimit=1  LowerLimit=-1
  Selector : Selector  InputPortWidth=3  IndexOptions=Index vector (dialog)  Indices=[ 3]  OutputSizes=1
  Selector1 : Selector  InputPortWidth=3  IndexOptions=Index vector (dialog)  Indices=1  OutputSizes=1
  Selector2 : Selector  InputPortWidth=3  IndexOptions=Index vector (dialog)  Indices=2  OutputSizes=1
  pitch_deadzone_inv : MATLAB Function  TreatAsAtomicUnit=on
  roll_deadzone_inv : MATLAB Function  TreatAsAtomicUnit=on
  yawrare_deadzone_inv : MATLAB Function  TreatAsAtomicUnit=on
  stabilizd_ref : Outport
  wires:
  Constant7/1 -> Data Type Conversion4/1  "CH5"
  Saturation4/1 -> Mux1/4  "r"
  Saturation1/1 -> Mux1/3  "z"
  Constant8/1 -> Data Type Conversion5/1  "CH7"
  Saturation2/1 -> Mux1/1  "x"
  Gain1/1 -> pitch_deadzone_inv/1(u)
  Selector2/1 -> Gain1/1
  Data Type Conversion5/1 -> Mux1/6  "CH7"
  euler_ref/1 -> Selector2/1, Selector1/1
  Gain10/1 -> roll_deadzone_inv/1(u)
  Selector/1 -> Gain12/1
  Mux1/1 -> stabilizd_ref/1  "rc"
  throttle/1 -> Saturation1/1  "CH2"
  Selector1/1 -> Gain10/1
  Data Type Conversion4/1 -> Mux1/5  "CH5"
  Gain12/1 -> yawrare_deadzone_inv/1(u)
  Saturation3/1 -> Mux1/2  "y"
  rates_r_ref/1 -> Selector/1
  roll_deadzone_inv/1(y) -> Saturation3/1
  yawrare_deadzone_inv/1(y) -> Saturation4/1
  pitch_deadzone_inv/1(y) -> Gain4/1
  Gain4/1 -> Saturation2/1

== system LW_ctrl_241029_1/Output/OutputSelect/Sim/Lifting Body Airframe/Estimator/Sensor Model/GPS/NoiseFilter1 ==
  In1 : Inport
  Demux : Demux  Outputs=3
  Mux1 : Mux  Inputs=3
  Transfer Fcn1 : TransferFcn  Denominator=[0.05 1]
  Transfer Fcn2 : TransferFcn  Denominator=[0.05 1]
  Transfer Fcn4 : TransferFcn  Denominator=[0.05 1]
  Out1 : Outport  VectorParamsAs1DForOutWhenUnconnected=off
  wires:
  Demux/2 -> Transfer Fcn1/1
  Transfer Fcn1/1 -> Mux1/2
  Demux/1 -> Transfer Fcn4/1
  Transfer Fcn2/1 -> Mux1/3
  Transfer Fcn4/1 -> Mux1/1
  Demux/3 -> Transfer Fcn2/1
  In1/1 -> Demux/1
  Mux1/1 -> Out1/1

== matlab function LW_ctrl_241029_1/Output/OutputSelect/HIL/MATLAB Function2 ==
  data: LW_LED parameter; LW_USE_SER parameter; LW_COOR_TURN parameter; LW_AERO_COM parameter; LW_TEST_EN parameter; LW_FEST_EN parameter; LW_F_MAP parameter; LW_REX_YAW parameter; LW_DMZ0 parameter; LW_DMZ_MIN parameter; LW_YAW_KAP parameter; LW_YAW_KAD parameter; LW_ANGLE parameter; LW_MASS parameter; LW_THR_HOVER parameter; LW_THR_LOW parameter; LW_DTHR parameter; LW_DSER parameter; LW_AERO_C0 parameter; LW_AERO_C1 parameter; LW_AERO_Y0 parameter; LW_LBCL_D parameter; LW_LBCM_D parameter; LW_OB_TYPE parameter; LW_FEST_WNXY parameter; LW_FEST_WNZ parameter; LW_FEST_SIGXY parameter; LW_FEST_SIGZ parameter; LW_FEST_LAMXY parameter; LW_FEST_LAMZ parameter; LW_FEST_P parameter; LW_FEST_DT parameter; LW_FEST_TDT parameter; LW_TEST_WNXY parameter; LW_TEST_WNZ parameter; LW_TEST_SIGXY parameter; LW_TEST_SIGZ parameter; LW_TEST_LAMXY parameter; LW_TEST_LAMZ parameter; LW_TEST_DTXY parameter; LW_TEST_DTZ parameter; LW_TEST_WBDT parameter; LW_TEST_TDT parameter; LW_VA_TMIN parameter; LW_VA_TMAX parameter; LW_MIXER_GAM parameter; LW_W_FZ parameter; LW_W_TAOX parameter; LW_W_TAOY parameter; LW_W_TAOZ parameter; LW_W_SER parameter; LW_W_SERH parameter; LW_SER_LP parameter; LW_MAN_ROLL_MAX parameter; LW_MAN_PITCH_MAX parameter; LW_WY_MAX parameter; LW_WY_DE_MAX parameter; LW_WX_MAX parameter; LW_WZ_MAX parameter; LW_ACRO_P_MAX parameter; LW_ACRO_R_MAX parameter; LW_ACRO_Y_MAX parameter; LW_PITCH_P parameter; LW_WY_P parameter; LW_WY_I parameter; LW_WY_D parameter; LW_WY_N parameter; LW_ROLL_P parameter; LW_WX_P parameter; LW_WX_I parameter; LW_WX_D parameter; LW_WX_N parameter; LW_YAW_P parameter; LW_WZ_P parameter; LW_WZ_I parameter; LW_WZ_D parameter; LW_WZ_N parameter; LW_WX_FF parameter; LW_WY_FF parameter; LW_WZ_FF parameter; LW_TAUXYSP_FZ parameter; LW_TAUXYSP_TM parameter; LW_TAUZSP_FZ parameter; LW_TAUZSP_TM parameter; LW_ACCSP_FZ parameter; LW_ACCSP_TM parameter; LW_TILTMAX_AIR parameter; LW_LAT_CIRCLE parameter; LW_X_VEL_MAX parameter; LW_X_ACCEL_MAX parameter; LW_X_ACCEL_MIN parameter; LW_X_JERK_MAX parameter; LW_Y_VEL_MAX parameter; LW_Y_ACCEL_MAX parameter; LW_Y_ACCEL_MIN parameter; LW_Y_JERK_MAX parameter; LW_Z_VEL_MAX_UP parameter; LW_Z_ACCEL_LOW parameter; LW_Z_ACCEL_UP parameter; LW_Z_JERK_MAX parameter; LW_VEL_DT parameter; LW_X_FF parameter; LW_Y_FF parameter; LW_Z_FF parameter; LW_X_P parameter; LW_X_VEL_P parameter; LW_X_VEL_I parameter; LW_X_VEL_D parameter; LW_X_VEL_N parameter; LW_Y_P parameter; LW_Y_VEL_P parameter; LW_Y_VEL_I parameter; LW_Y_VEL_D parameter; LW_Y_VEL_N parameter; LW_Z_P parameter; LW_Z_VEL_P parameter; LW_Z_VEL_I parameter; LW_Z_VEL_D parameter; LW_Z_VEL_N parameter; LW_ACCX_FF parameter; LW_ACCY_FF parameter; LW_ACCZ_FF parameter; LW_OB_CIRCLE_R parameter; LW_OB_CIRCLE_V parameter; LW_OB_CIRCLE_W parameter; RC1_MIN parameter; RC1_MAX parameter; RC1_REV parameter; RC2_MIN parameter; RC2_MAX parameter; RC2_REV parameter; RC3_MIN parameter; RC3_MAX parameter; RC3_REV parameter; RC4_MIN parameter; RC4_MAX parameter; RC4_REV parameter; LW_MAN_ROLL_DZ parameter; LW_MAN_PITCH_DZ parameter; LW_MAN_WX_DZ parameter; LW_MAN_WY_DZ parameter; LW_MAN_WZ_DZ parameter; LW_X_VEL_DZ parameter; LW_Y_VEL_DZ parameter; LW_Z_VEL_DZ parameter; LW_SERVOR_REV parameter; LW_SERVOL_REV parameter; LW_SERVOR_MAX parameter; LW_SERVOR_MIN parameter; LW_SERVOL_MAX parameter; LW_SERVOL_MIN parameter; LW_SERVOR_CON parameter; out output
function out  = yourFcn( ...
LW_LED, LW_USE_SER, LW_COOR_TURN, LW_AERO_COM, LW_TEST_EN, LW_FEST_EN, LW_F_MAP, LW_REX_YAW, ...
LW_DMZ0, LW_DMZ_MIN, LW_YAW_KAP, LW_YAW_KAD, LW_ANGLE, ...
LW_MASS, LW_THR_HOVER, LW_THR_LOW, LW_DTHR, LW_DSER, LW_AERO_C0, LW_AERO_C1, LW_AERO_Y0, LW_LBCL_D, LW_LBCM_D, LW_OB_TYPE, ...
LW_FEST_WNXY, LW_FEST_WNZ, LW_FEST_SIGXY, LW_FEST_SIGZ, LW_FEST_LAMXY, LW_FEST_LAMZ, LW_FEST_P, LW_FEST_DT, LW_FEST_TDT, ...
LW_TEST_WNXY, LW_TEST_WNZ, LW_TEST_SIGXY, LW_TEST_SIGZ, LW_TEST_LAMXY, LW_TEST_LAMZ, LW_TEST_DTXY, LW_TEST_DTZ, LW_TEST_WBDT, LW_TEST_TDT, ...
LW_VA_TMIN, LW_VA_TMAX, LW_MIXER_GAM, LW_W_FZ, LW_W_TAOX, LW_W_TAOY, LW_W_TAOZ, LW_W_SER, LW_W_SERH, LW_SER_LP, ...
LW_MAN_ROLL_MAX, LW_MAN_PITCH_MAX, LW_WY_MAX, LW_WY_DE_MAX, LW_WX_MAX, LW_WZ_MAX, LW_ACRO_P_MAX, LW_ACRO_R_MAX, LW_ACRO_Y_MAX, ...
LW_PITCH_P, LW_WY_P, LW_WY_I, LW_WY_D, LW_WY_N, LW_ROLL_P, LW_WX_P, LW_WX_I, LW_WX_D, LW_WX_N, LW_YAW_P, LW_WZ_P, LW_WZ_I, LW_WZ_D, LW_WZ_N, ...
LW_WX_FF, LW_WY_FF, LW_WZ_FF, LW_TAUXYSP_FZ, LW_TAUXYSP_TM, LW_TAUZSP_FZ, LW_TAUZSP_TM, LW_ACCSP_FZ, LW_ACCSP_TM, ...
LW_TILTMAX_AIR, LW_LAT_CIRCLE, LW_X_VEL_MAX, LW_X_ACCEL_MAX, LW_X_ACCEL_MIN, LW_X_JERK_MAX, LW_Y_VEL_MAX, LW_Y_ACCEL_MAX, LW_Y_ACCEL_MIN, LW_Y_JERK_MAX, ...
LW_Z_VEL_MAX_UP, LW_Z_ACCEL_LOW, LW_Z_ACCEL_UP, LW_Z_JERK_MAX, LW_VEL_DT, ...
LW_X_FF, LW_Y_FF, LW_Z_FF, LW_X_P, LW_X_VEL_P, LW_X_VEL_I, LW_X_VEL_D, LW_X_VEL_N, LW_Y_P, LW_Y_VEL_P, LW_Y_VEL_I, LW_Y_VEL_D, LW_Y_VEL_N, ...
LW_Z_P, LW_Z_VEL_P, LW_Z_VEL_I, LW_Z_VEL_D, LW_Z_VEL_N, LW_ACCX_FF, LW_ACCY_FF, LW_ACCZ_FF, ...
LW_OB_CIRCLE_R, LW_OB_CIRCLE_V, LW_OB_CIRCLE_W, ...
RC1_MIN, RC1_MAX, RC1_REV, RC2_MIN, RC2_MAX, RC2_REV, RC3_MIN, RC3_MAX, RC3_REV, RC4_MIN, RC4_MAX, RC4_REV, ...
LW_MAN_ROLL_DZ, LW_MAN_PITCH_DZ, LW_MAN_WX_DZ, LW_MAN_WY_DZ, LW_MAN_WZ_DZ, LW_X_VEL_DZ, LW_Y_VEL_DZ, LW_Z_VEL_DZ, ...
LW_SERVOR_REV, LW_SERVOL_REV, LW_SERVOR_MAX, LW_SERVOR_MIN, LW_SERVOL_MAX, LW_SERVOL_MIN, LW_SERVOR_CON)


out = LW_SERVOR_REV;
end

== matlab function LW_ctrl_241029_1/Output/OutputSelect/HIL/MATLAB Function ==
  data: u input; y output
function y = fcn(u)

if u > 1700 
    y = boolean(1);
else
    y = boolean(0);
end

== matlab function LW_ctrl_241029_1/Output/OutputSelect/HIL/MATLAB Function1 ==
  data: u input; y output
function y = fcn(u)

t = u(4);
u(4) = u(2);
u(2) = t;
y = u;

== matlab function LW_ctrl_241029_1/Output/OutputSelect/Sim/nan_inf ==
  data: u input; y output
function y = fcn(u)

for i = 1:length(u)
    if isnan(u(i)) || isinf(u(i))
        if i > 4
            u(i) = 1500;
        else
            u(i) = 1000;
        end
    end
end
y = u;

== matlab function LW_ctrl_241029_1/Controller/PID_Controller/PID_Controller/nan_inf_mode ==
  data: u input; y output
function y = fcn(u)
for i = 1:length(u)
    if isnan(u(i)) || isinf(u(i))
        u(i) = ControlMode.DISARM;
    end
end
y = u;

== matlab function LW_ctrl_241029_1/Controller/PID_Controller/PID_Controller/toPWM/toPWM ==
  data: w input; pwm output; ModelParam_motorUp1 parameter; ModelParam_motorUp2 parameter; ModelParam_motorUp3 parameter; voltage input; batt_connected input
function pwm = fcn(w, ModelParam_motorUp1, ModelParam_motorUp2, ModelParam_motorUp3, voltage, batt_connected)
a = ModelParam_motorUp1;
b = ModelParam_motorUp2;
sigma = zeros(4,1);
if batt_connected 
    % 4S
    if voltage < 12.0
        voltage = single(12.0);
    elseif voltage > 17
        voltage = single(17.0);
    end
else
    voltage = single(16.0);
end

for i = 1:4
    c = ModelParam_motorUp3 - w(i);
    if a ~= 0
        sigma(i) = (-b+sqrt(abs(b^2-4*a*c)))/(2*a)/voltage;
    else
        sigma(i) = -c/ModelParam_motorUp2/voltage;
    end
end
   
if sigma(i) < -0.2 
    sigma(i) = -0.2;
elseif sigma(i) > 1
    sigma(i) = 1;
end
pwm = single(sigma*1000 + 1000);

== matlab function LW_ctrl_241029_1/Controller/PID_Controller/PID_Controller/local_pos_ref_selector/nan_inf_mode ==
  data: u input; y output
function y = fcn(u)

for i = 1:length(u)
    if isnan(u(i)) || isinf(u(i))
        u(i) = ControlMode.DISARM;
    end
end
y = u;

== matlab function LW_ctrl_241029_1/navigator/navigator_manual/f1 ==
  data: in input; y output; hover input
function y = thr_curve(in, hover)
%Function description:
%  throttle curve. When the throttle is in the middle position, the output
%  is hovering throttle value.
%Input:
%  in: normalized throttle, range from 0 to 1
%  hover: hovering throttle value
%Output:
%  y: processed throttle value
if in < 0.5
	y=2 * in * hover;
else
	y=hover + 2 * (in - 0.5) * (1.0 - hover);
end

== matlab function LW_ctrl_241029_1/Controller/PID_Controller/PID_Controller/local_pos_ref_selector/nan_inf_mode1 ==
  data: u input; y output
function y = fcn(u)

for i = 1:length(u)
    if isnan(u(i)) || isinf(u(i))
        u(i) = FlightMode.PILOT;
    end
end
y = u;
